simulink model "azfuzzy"  (R2020b)
settings: Solver=VariableStepAuto  StartTime=0.0  StopTime=100.0  RelTol=1e-3
libraries: fuzblock x1
settings Model: Creator=admin  LastModifiedBy=admin

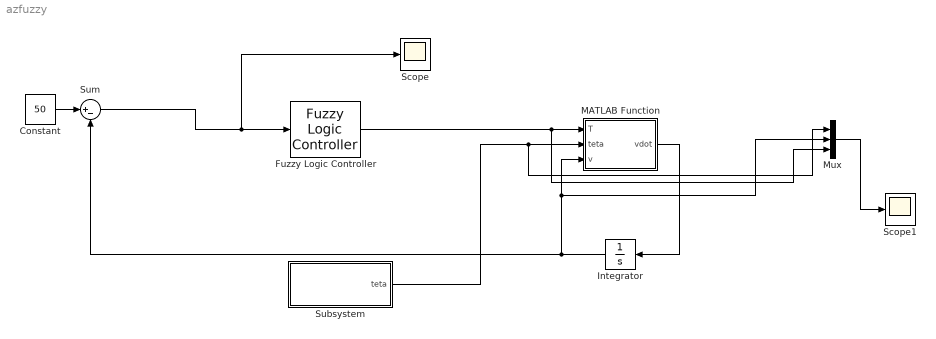
== system azfuzzy ==
  Constant : Constant  Value=50
  Fuzzy Logic Controller : fuzblock/Fuzzy Logic  Controller  FIS='fuzzylogic.fis'  OutputSampleNumber=101  DataType=double  FuzzifiedInputs=off  RuleFiringStrengths=off  RuleOutputs=off  AggregatedOutputs=off  SimulateUsing=Interpreted execution  OutOfRangeInputValueMessage=warning  NoRuleFiredMessage=warning  EmptyOutputFuzzySetMessage=warning
  Integrator : Integrator  InitialCondition=zeros(1,1)
  MATLAB Function : MATLAB Function  TreatAsAtomicUnit=on
  Mux : Mux  Inputs=3
  Scope : Scope
  Scope1 : Scope
  Subsystem : Subsystem
  Sum : Sum  Inputs=|+-
  wires:
  MATLAB Function/1(vdot) -> Integrator/1
  Integrator/1 -> Sum/2, Mux/2, MATLAB Function/3(v)
  Subsystem/1(teta) -> Mux/1, MATLAB Function/2(teta)
  Fuzzy Logic Controller/1 -> Mux/3, MATLAB Function/1(T)
  Sum/1 -> Scope/1, Fuzzy Logic Controller/1
  Constant/1 -> Sum/1
  Mux/1 -> Scope1/1

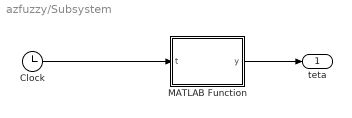
== system azfuzzy/Subsystem ==
  Clock : Clock
      settings: Decimation=100
  MATLAB Function : MATLAB Function  TreatAsAtomicUnit=on
  teta : Outport
  wires:
  MATLAB Function/1(y) -> teta/1
  Clock/1 -> MATLAB Function/1(t)

== matlab function azfuzzy/MATLAB Function ==
  data: T input; vdot output; teta input; v input
function vdot = fcn(T,teta,v)
vdot=zeros(1,1)
A=[-0.1]
B=[1 0.1]
source=[T;teta]
vdot = A*v+B*source
end

== matlab function azfuzzy/Subsystem/MATLAB Function ==
  data: t input; y output
function y = fcn(t)
if (0<t&&t<20)
    y = (t/4)-5
elseif(t>=20&&t<=40)
    y=0
elseif(t>40&&t<80)
    y=(t/4)-10
else
    y=10
end
end
